simulink model "Class_Project_Problem6_simulink_FILE"  (R2025b)
settings: Solver=VariableStepAuto  StartTime=0.0  StopTime=10.0  RelTol=1e-3
undefined symbols (not defined in the file): c, F, k, m
settings Model: Creator=benja  LastModifiedBy=benja

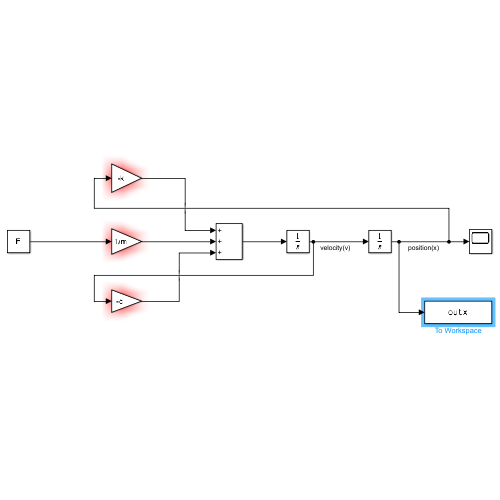
[thumbnail: Simulink's stored preview of the top-level diagram]
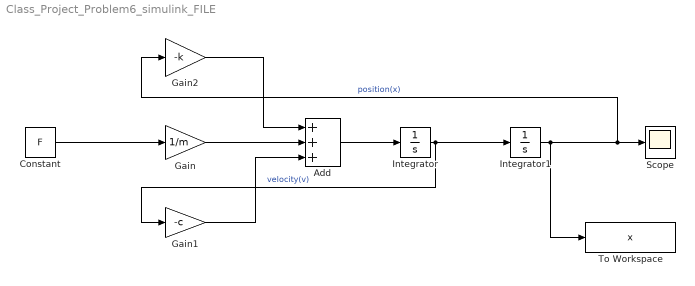
== system Class_Project_Problem6_simulink_FILE ==
  Add : Sum  Inputs=+++
  Constant : Constant  Value=F
  Gain : Gain  Gain=1/m
  Gain1 : Gain  Gain=-c
  Gain2 : Gain  Gain=-k
  Integrator : Integrator
  Integrator1 : Integrator  InitialCondition=5
  Scope : Scope
  To Workspace : ToWorkspace  VariableName=x  SampleTime=-1
  wires:
  Gain2/1 -> Add/1
  Gain/1 -> Add/2
  Gain1/1 -> Add/3
  Add/1 -> Integrator/1
  Integrator/1 -> Gain1/1, Integrator1/1  "velocity(v)"
  Integrator1/1 -> To Workspace/1, Gain2/1, Scope/1  "position(x)"
  Constant/1 -> Gain/1
